simulink model "ScriptDemo"  (R2022b)
settings: configuration reference "TmVcThermal_Configuration_sub" (kept outside this file)
undefined symbols (not defined in the file): aaaa, bbbb, cTmComprCtrl_D_u8HvacFlowTable_db, cTmComprCtrl_D_u8HvacFlowTable_sw, cTmComprCtrl_n_i16ChillCmpIMax, cTmComprCtrl_n_i16ChillCmpIMin, cTmComprCtrl_n_i16ChillCmpIMin666, cTmComprCtrl_n_i16ChillCmpPMax, cTmComprCtrl_n_i16ChillCmpPMin, cTmComprCtrl_n_i16CmpChillCoolRpmKiMax, cTmComprCtrl_n_i16CmpChillCoolRpmKiMin, cTmComprCtrl_n_i16CmpChillCoolRpmKpMax, cTmComprCtrl_n_i16CmpChillCoolRpmKpMin, cTmComprCtrl_n_i16CmpCoolRpmKiMax, cTmComprCtrl_n_i16CmpCoolRpmKiMin, cTmComprCtrl_n_i16CmpCoolRpmKpMax, cTmComprCtrl_n_i16CmpCoolRpmKpMin, cTmComprCtrl_n_i16SM4CmpHeatKiMax, cTmComprCtrl_n_i16SM4CmpHeatKiMin, cTmComprCtrl_n_i16SM4CmpHeatKpMax, cTmComprCtrl_n_i16SM4CmpHeatKpMin, cTmComprCtrl_n_i16SM5CmpHeatKiMax, cTmComprCtrl_n_i16SM5CmpHeatKiMin, cTmComprCtrl_n_i16SM5CmpHeatKpMax, cTmComprCtrl_n_i16SM5CmpHeatKpMin, cTmComprCtrl_n_i16SM6CmpHeatKiMax, cTmComprCtrl_n_i16SM6CmpHeatKiMin, cTmComprCtrl_n_i16SM6CmpHeatKpMax, cTmComprCtrl_n_i16SM6CmpHeatKpMin, cTmComprCtrl_n_u16CmpMaxSpdFanFltLimt, cTmComprCtrl_n_u16CmpMaxSpdLoSidePFltLimt, cTmComprCtrl_n_u16CmpMaxSpdSensorFltLimt, cTmComprCtrl_n_u16CompMinRpm, cTmComprCtrl_n_u16CompRpmIncThres, cTmComprCtrl_t_u16BattCooltFFPeriod, cTmComprCtrl_t_u16BattCooltPIPeriod, cTmComprCtrl_t_u16CmpCoolFFPeriod, cTmComprCtrl_t_u16CmpCoolPIPeriod, cTmComprCtrl_t_u16CoolCmpChillFFPeriod, cTmComprCtrl_t_u16CoolCmpChillPIPeriod, cTmComprCtrl_t_u16SM4CmpHeatFFPeriod, cTmComprCtrl_t_u16SM4CmpHeatPIPeriod, cTmComprCtrl_t_u16SM5CmpHeatFFPeriod, cTmComprCtrl_t_u16SM5CmpHeatPIPeriod, cTmComprCtrl_t_u16SM6CmpHeatFFPeriod, cTmComprCtrl_t_u16SM6CmpHeatPIPeriod, cTmComprCtrl_Te_EvapClearInteg, cTmComprCtrl_Te_i16HpReqTempSaturoffset, cTmComprCtrl_Te_i16SatLpReplaceDiff, cTmComprCtrl_Te_i16SM3BatDiffStartEvapDecOffset, cTmComprCtrl_Te_i16SM3EvapLo, cTmComprCtrl_Te_i16SM3TBatDiffEntEvapDecOffset, cTmComprCtrl_Te_i16SM3TBatDiffEntEvapDecOffsetQuit, cTmComprCtrl_Te_s32ErrCmpChillPIContinueCoolH, cTmComprCtrl_Te_s32ErrCmpChillPIContinueCoolL, cTmComprCtrl_Te_s32ErrCmpPIContinueChillH, cTmComprCtrl_Te_s32ErrCmpPIContinueChillL, cTmComprCtrl_Te_s32ErrCmpPIContinueCoolH, cTmComprCtrl_Te_s32ErrCmpPIContinueCoolL, cTmComprCtrl_Te_s32ErrCmpPIContinueHeatH ... (+398)
libraries: simulink x782, PCMULib x640, simulink_need_slupdate x4
(part 12 of 41)

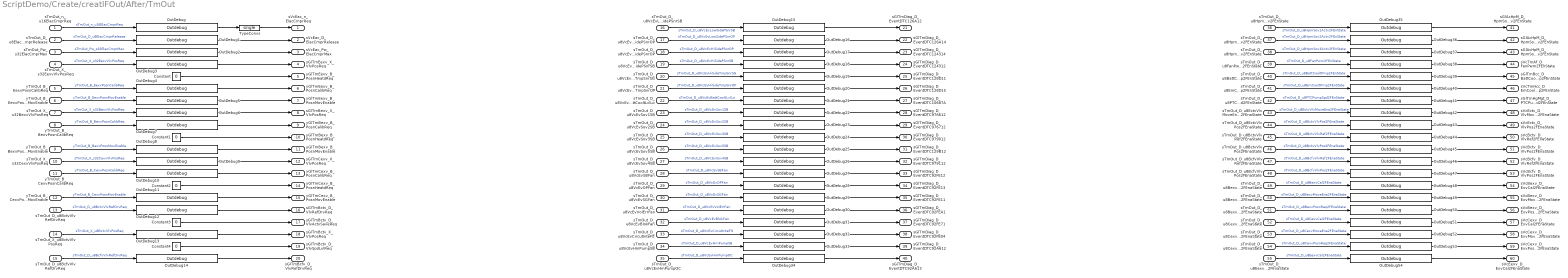
== system ScriptDemo/Create/creatIFOut/After/TmOut ==
  sTmOut_n_u16ElacCmprReq : Inport  OutDataTypeStr=uint16
  sTmOut_D_u8ElacCmprRelease : Inport  Port=2  OutDataTypeStr=uint8
  sTmOut_Pw_s32ElacCmprMax : Inport  Port=3  OutDataTypeStr=single
  sTmOut_X_s32EexvVlvPosReq : Inport  Port=4  OutDataTypeStr=single
  yTmOut_B_EexvPosnCalibReq : Inport  Port=5  OutDataTypeStr=boolean
  yTmOut_B_EexvPosnMovEnable : Inport  Port=6  OutDataTypeStr=boolean
  sTmOut_X_s32BexvVlvPosReq : Inport  Port=7  OutDataTypeStr=single
  yTmOut_B_BexvPosnCalibReq : Inport  Port=8  OutDataTypeStr=boolean
  yTmOut_B_BexvPosnMovEnable : Inport  Port=9  OutDataTypeStr=boolean
  sTmOut_X_s32CexvVlvPosReq : Inport  Port=10  OutDataTypeStr=single
  yTmOut_B_CexvPosnCalibReq : Inport  Port=11  OutDataTypeStr=boolean
  yTmOut_B_CexvPosnMovEnable : Inport  Port=12  OutDataTypeStr=boolean
  sTmOut_D_u8BctvVlvRefDrvReq : Inport  Port=13  OutDataTypeStr=uint8
  sTmOut_X_u8BctvVlvPosReq : Inport  Port=14  OutDataTypeStr=uint8
  sTmOut_D_u8BcfvVlvRefDrvReq : Inport  Port=15  OutDataTypeStr=uint8
  sTmOut_D_u8VcEvLowSidePSnrSB : Inport  Port=16  OutDataTypeStr=uint8
  sTmOut_D_u8VcEvLowSidePSnrOP : Inport  Port=17  OutDataTypeStr=uint8
  sTmOut_D_u8VcEvHiSidePSnrOP : Inport  Port=18  OutDataTypeStr=uint8
  sTmOut_D_u8VcEvHiSidePSnrSB : Inport  Port=19  OutDataTypeStr=uint8
  sTmOut_D_u8VcEvHiSideTmpSnrSG : Inport  Port=20  OutDataTypeStr=uint8
  sTmOut_D_u8VcEvHiSideTmpSnrOP : Inport  Port=21  OutDataTypeStr=uint8
  sTmOut_D_u8VcEvBattCooltLvlLo : Inport  Port=22  OutDataTypeStr=uint8
  sTmOut_D_u8VcEvSov1SB : Inport  Port=23  OutDataTypeStr=uint8
  sTmOut_D_u8VcEvSov2SB : Inport  Port=24  OutDataTypeStr=uint8
  sTmOut_D_u8VcEvSov3SB : Inport  Port=25  OutDataTypeStr=uint8
  sTmOut_D_u8VcEvSov5SB : Inport  Port=26  OutDataTypeStr=uint8
  sTmOut_D_u8VcEvSov4SB : Inport  Port=27  OutDataTypeStr=uint8
  sTmOut_D_u8VcEvSBFan : Inport  Port=28  OutDataTypeStr=uint8
  sTmOut_D_u8VcEvOPFan : Inport  Port=29  OutDataTypeStr=uint8
  sTmOut_D_u8VcEvSGFan : Inport  Port=30  OutDataTypeStr=uint8
  sTmOut_D_u8VcEvVolErrFan : Inport  Port=31  OutDataTypeStr=uint8
  sTmOut_D_u8VcEvBlokFan : Inport  Port=32  OutDataTypeStr=uint8
  sTmOut_D_u8VcEvCircutInteFlt : Inport  Port=33  OutDataTypeStr=uint8
  sTmOut_D_u8VcEvHmPumpSB : Inport  Port=34  OutDataTypeStr=uint8
  sTmOut_D_u8VcEvHmPumpOC : Inport  Port=35  OutDataTypeStr=uint8
  sTmOut_D_u8HpmSov1Actv2FEnState : Inport  Port=36  OutDataTypeStr=uint8
  sTmOut_D_u8HpmSov2Actv2FEnState : Inport  Port=37  OutDataTypeStr=uint8
  sTmOut_D_u8HpmSov3Actv2FEnState : Inport  Port=38  OutDataTypeStr=uint8
  sTmOut_D_u8FanPwm2FEnState : Inport  Port=39  OutDataTypeStr=uint8
  sTmOut_D_u8BattCooltPmp2FEnState : Inport  Port=40  OutDataTypeStr=uint8
  sTmOut_D_u8EmCooltPmp2FEnState : Inport  Port=41  OutDataTypeStr=uint8
  sTmOut_D_u8PTCPumpSpd2FEnState : Inport  Port=42  OutDataTypeStr=uint8
  sTmOut_D_u8EctvVlvMoveEna2FEnaState : Inport  Port=43  OutDataTypeStr=uint8
  sTmOut_D_u8EctvVlvPos2FEnaState : Inport  Port=44  OutDataTypeStr=uint8
  sTmOut_D_u8BctvVlvRef2FEnaState : Inport  Port=45  OutDataTypeStr=uint8
  sTmOut_D_u8BctvVlvPos2FEnaState : Inport  Port=46  OutDataTypeStr=uint8
  sTmOut_D_u8BcfvVlvRef2FEnaState : Inport  Port=47  OutDataTypeStr=uint8
  sTmOut_D_u8BcfvVlvPos2FEnaState : Inport  Port=48  OutDataTypeStr=uint8
  sTmOut_D_u8BexvCal2FEnaState : Inport  Port=49  OutDataTypeStr=uint8
  sTmOut_D_u8BexvMoveEna2FEnaState : Inport  Port=50  OutDataTypeStr=uint8
  sTmOut_D_u8BexvPosnReq2FEnaState : Inport  Port=51  OutDataTypeStr=uint8
  sTmOut_D_u8CexvCal2FEnaState : Inport  Port=52  OutDataTypeStr=uint8
  sTmOut_D_u8CexvMoveEna2FEnaState : Inport  Port=53  OutDataTypeStr=uint8
  sTmOut_D_u8CexvPosnReq2FEnaState : Inport  Port=54  OutDataTypeStr=uint8
  sTmOut_D_u8EexvCal2FEnaState : Inport  Port=55  OutDataTypeStr=uint8
  Constant : Constant  Value=0  OutDataTypeStr=boolean
  Constant1 : Constant  Value=0  OutDataTypeStr=boolean
  Constant2 : Constant  Value=0  OutDataTypeStr=boolean
  Constant3 : Constant  Value=0  OutDataTypeStr=uint8
  Constant4 : Constant  Value=0  OutDataTypeStr=uint8
  OutDebug : PCMULib/Interface/Outdebug  SWI=cTmOut_n_u16ElacCmprReq_sw  DBI=cTmOut_n_u16ElacCmprReq_db
      settings: SourceProductName=PCMULib
  OutDebug1 : PCMULib/Interface/Outdebug  SWI=cTmOut_D_u8ElacCmprRelease_sw  DBI=cTmOut_D_u8ElacCmprRelease_db
      settings: SourceProductName=PCMULib
  OutDebug10 : PCMULib/Interface/Outdebug  SWI=cTmOut_B_CexvPosnCalibReq_sw  DBI=cTmOut_B_CexvPosnCalibReq_db
      settings: SourceProductName=PCMULib
  OutDebug11 : PCMULib/Interface/Outdebug  SWI=cTmOut_B_CexvPosnMovEnable_sw  DBI=cTmOut_B_CexvPosnMovEnable_db
      settings: SourceProductName=PCMULib
  OutDebug12 : PCMULib/Interface/Outdebug  SWI=cTmOut_D_u8BctvVlvRefDrvReq_sw  DBI=cTmOut_D_u8BctvVlvRefDrvReq_db
      settings: SourceProductName=PCMULib
  OutDebug13 : PCMULib/Interface/Outdebug  SWI=cTmOut_X_u8BctvVlvPosReq_sw  DBI=cTmOut_X_u8BctvVlvPosReq_db
      settings: SourceProductName=PCMULib
  OutDebug14 : PCMULib/Interface/Outdebug  SWI=cTmOut_D_u8BcfvVlvRefDrvReq_sw  DBI=cTmOut_D_u8BcfvVlvRefDrvReq_db
      settings: SourceProductName=PCMULib
  OutDebug15 : PCMULib/Interface/Outdebug  SWI=cTmOut_D_u8VcEvLowSidePSnrSB_sw  DBI=cTmOut_D_u8VcEvLowSidePSnrSB_db
      settings: SourceProductName=PCMULib
  OutDebug16 : PCMULib/Interface/Outdebug  SWI=cTmOut_D_u8VcEvLowSidePSnrOP_sw  DBI=cTmOut_D_u8VcEvLowSidePSnrOP_db
      settings: SourceProductName=PCMULib
  OutDebug17 : PCMULib/Interface/Outdebug  SWI=cTmOut_D_u8VcEvHiSidePSnrOP_sw  DBI=cTmOut_D_u8VcEvHiSidePSnrOP_db
      settings: SourceProductName=PCMULib
  OutDebug18 : PCMULib/Interface/Outdebug  SWI=cTmOut_D_u8VcEvHiSidePSnrSB_sw  DBI=cTmOut_D_u8VcEvHiSidePSnrSB_db
      settings: SourceProductName=PCMULib
  OutDebug19 : PCMULib/Interface/Outdebug  SWI=cTmOut_D_u8VcEvHiSideTmpSnrSG_sw  DBI=cTmOut_D_u8VcEvHiSideTmpSnrSG_db
      settings: SourceProductName=PCMULib
  OutDebug2 : PCMULib/Interface/Outdebug  SWI=cTmOut_Pw_s32ElacCmprMax_sw  DBI=cTmOut_Pw_s32ElacCmprMax_db
      settings: SourceProductName=PCMULib
  OutDebug20 : PCMULib/Interface/Outdebug  SWI=cTmOut_D_u8VcEvHiSideTmpSnrOP_sw  DBI=cTmOut_D_u8VcEvHiSideTmpSnrOP_db
      settings: SourceProductName=PCMULib
  OutDebug21 : PCMULib/Interface/Outdebug  SWI=cTmOut_D_u8VcEvBattCooltLvlLo_sw  DBI=cTmOut_D_u8VcEvBattCooltLvlLo_db
      settings: SourceProductName=PCMULib
  OutDebug22 : PCMULib/Interface/Outdebug  SWI=cTmOut_D_u8VcEvSov1SB_sw  DBI=cTmOut_D_u8VcEvSov1SB_db
      settings: SourceProductName=PCMULib
  OutDebug23 : PCMULib/Interface/Outdebug  SWI=cTmOut_D_u8VcEvSov2SB_sw  DBI=cTmOut_D_u8VcEvSov2SB_db
      settings: SourceProductName=PCMULib
  OutDebug24 : PCMULib/Interface/Outdebug  SWI=cTmOut_D_u8VcEvSov3SB_sw  DBI=cTmOut_D_u8VcEvSov3SB_db
      settings: SourceProductName=PCMULib
  OutDebug25 : PCMULib/Interface/Outdebug  SWI=cTmOut_D_u8VcEvSov5SB_sw  DBI=cTmOut_D_u8VcEvSov5SB_db
      settings: SourceProductName=PCMULib
  OutDebug26 : PCMULib/Interface/Outdebug  SWI=cTmOut_D_u8VcEvSov4SB_sw  DBI=cTmOut_D_u8VcEvSov4SB_db
      settings: SourceProductName=PCMULib
  OutDebug27 : PCMULib/Interface/Outdebug  SWI=cTmOut_D_u8VcEvSBFan_sw  DBI=cTmOut_D_u8VcEvSBFan_db
      settings: SourceProductName=PCMULib
  OutDebug28 : PCMULib/Interface/Outdebug  SWI=cTmOut_D_u8VcEvOPFan_sw  DBI=cTmOut_D_u8VcEvOPFan_db
      settings: SourceProductName=PCMULib
  OutDebug29 : PCMULib/Interface/Outdebug  SWI=cTmOut_D_u8VcEvSGFan_sw  DBI=cTmOut_D_u8VcEvSGFan_db
      settings: SourceProductName=PCMULib
  OutDebug3 : PCMULib/Interface/Outdebug  SWI=cTmOut_X_s32EexvVlvPosReq_sw  DBI=cTmOut_X_s32EexvVlvPosReq_db
      settings: SourceProductName=PCMULib
  OutDebug30 : PCMULib/Interface/Outdebug  SWI=cTmOut_D_u8VcEvVolErrFan_sw  DBI=cTmOut_D_u8VcEvVolErrFan_db
      settings: SourceProductName=PCMULib
  OutDebug31 : PCMULib/Interface/Outdebug  SWI=cTmOut_D_u8VcEvBlokFan_sw  DBI=cTmOut_D_u8VcEvBlokFan_db
      settings: SourceProductName=PCMULib
  OutDebug32 : PCMULib/Interface/Outdebug  SWI=cTmOut_D_u8VcEvCircutInteFlt_sw  DBI=cTmOut_D_u8VcEvCircutInteFlt_db
      settings: SourceProductName=PCMULib
  OutDebug33 : PCMULib/Interface/Outdebug  SWI=cTmOut_D_u8VcEvHmPumpSB_sw  DBI=cTmOut_D_u8VcEvHmPumpSB_db
      settings: SourceProductName=PCMULib
  OutDebug34 : PCMULib/Interface/Outdebug  SWI=cTmOut_D_u8VcEvHmPumpOC_sw  DBI=cTmOut_D_u8VcEvHmPumpOC_db
      settings: SourceProductName=PCMULib
  OutDebug35 : PCMULib/Interface/Outdebug  SWI=cTmOut_D_u8HpmSov1Actv2FEnState_sw  DBI=cTmOut_D_u8HpmSov1Actv2FEnState_db
      settings: SourceProductName=PCMULib
  OutDebug36 : PCMULib/Interface/Outdebug  SWI=cTmOut_D_u8HpmSov2Actv2FEnState_sw  DBI=cTmOut_D_u8HpmSov2Actv2FEnState_db
      settings: SourceProductName=PCMULib
  OutDebug37 : PCMULib/Interface/Outdebug  SWI=cTmOut_D_u8HpmSov3Actv2FEnState_sw  DBI=cTmOut_D_u8HpmSov3Actv2FEnState_db
      settings: SourceProductName=PCMULib
  OutDebug38 : PCMULib/Interface/Outdebug  SWI=cTmOut_D_u8FanPwm2FEnState_sw  DBI=cTmOut_D_u8FanPwm2FEnState_db
      settings: SourceProductName=PCMULib
  OutDebug39 : PCMULib/Interface/Outdebug  SWI=cTmOut_D_u8BattCooltPmp2FEnState_sw  DBI=cTmOut_D_u8BattCooltPmp2FEnState_db
      settings: SourceProductName=PCMULib
  OutDebug4 : PCMULib/Interface/Outdebug  SWI=cTmOut_B_EexvPosnCalibReq_sw  DBI=cTmOut_B_EexvPosnCalibReq_db
      settings: SourceProductName=PCMULib
  OutDebug40 : PCMULib/Interface/Outdebug  SWI=cTmOut_D_u8EmCooltPmp2FEnState_sw  DBI=cTmOut_D_u8EmCooltPmp2FEnState_db
      settings: SourceProductName=PCMULib
  OutDebug41 : PCMULib/Interface/Outdebug  SWI=cTmOut_D_u8PTCPumpSpd2FEnState_sw  DBI=cTmOut_D_u8PTCPumpSpd2FEnState_db
      settings: SourceProductName=PCMULib
  OutDebug42 : PCMULib/Interface/Outdebug  SWI=cTmOut_D_u8EctvVlvMoveEna2FEnaState_sw  DBI=cTmOut_D_u8EctvVlvMoveEna2FEnaState_db
      settings: SourceProductName=PCMULib
  OutDebug43 : PCMULib/Interface/Outdebug  SWI=cTmOut_D_u8EctvVlvPos2FEnaState_sw  DBI=cTmOut_D_u8EctvVlvPos2FEnaState_db
      settings: SourceProductName=PCMULib
  OutDebug44 : PCMULib/Interface/Outdebug  SWI=cTmOut_D_u8BctvVlvRef2FEnaState_sw  DBI=cTmOut_D_u8BctvVlvRef2FEnaState_db
      settings: SourceProductName=PCMULib
  OutDebug45 : PCMULib/Interface/Outdebug  SWI=cTmOut_D_u8BctvVlvPos2FEnaState_sw  DBI=cTmOut_D_u8BctvVlvPos2FEnaState_db
      settings: SourceProductName=PCMULib
  OutDebug46 : PCMULib/Interface/Outdebug  SWI=cTmOut_D_u8BcfvVlvRef2FEnaState_sw  DBI=cTmOut_D_u8BcfvVlvRef2FEnaState_db
      settings: SourceProductName=PCMULib
  OutDebug47 : PCMULib/Interface/Outdebug  SWI=cTmOut_D_u8BcfvVlvPos2FEnaState_sw  DBI=cTmOut_D_u8BcfvVlvPos2FEnaState_db
      settings: SourceProductName=PCMULib
  OutDebug48 : PCMULib/Interface/Outdebug  SWI=cTmOut_D_u8BexvCal2FEnaState_sw  DBI=cTmOut_D_u8BexvCal2FEnaState_db
      settings: SourceProductName=PCMULib
  OutDebug49 : PCMULib/Interface/Outdebug  SWI=cTmOut_D_u8BexvMoveEna2FEnaState_sw  DBI=cTmOut_D_u8BexvMoveEna2FEnaState_db
      settings: SourceProductName=PCMULib
  OutDebug5 : PCMULib/Interface/Outdebug  SWI=cTmOut_B_EexvPosnMovEnable_sw  DBI=cTmOut_B_EexvPosnMovEnable_db
      settings: SourceProductName=PCMULib
  OutDebug50 : PCMULib/Interface/Outdebug  SWI=cTmOut_D_u8BexvPosnReq2FEnaState_sw  DBI=cTmOut_D_u8BexvPosnReq2FEnaState_db
      settings: SourceProductName=PCMULib
  OutDebug51 : PCMULib/Interface/Outdebug  SWI=cTmOut_D_u8CexvCal2FEnaState_sw  DBI=cTmOut_D_u8CexvCal2FEnaState_db
      settings: SourceProductName=PCMULib
  OutDebug52 : PCMULib/Interface/Outdebug  SWI=cTmOut_D_u8CexvMoveEna2FEnaState_sw  DBI=cTmOut_D_u8CexvMoveEna2FEnaState_db
      settings: SourceProductName=PCMULib
  OutDebug53 : PCMULib/Interface/Outdebug  SWI=cTmOut_D_u8CexvPosnReq2FEnaState_sw  DBI=cTmOut_D_u8CexvPosnReq2FEnaState_db
      settings: SourceProductName=PCMULib
  OutDebug54 : PCMULib/Interface/Outdebug  SWI=cTmOut_D_u8EexvCal2FEnaState_sw  DBI=cTmOut_D_u8EexvCal2FEnaState_db
      settings: SourceProductName=PCMULib
  OutDebug6 : PCMULib/Interface/Outdebug  SWI=cTmOut_X_s32BexvVlvPosReq_sw  DBI=cTmOut_X_s32BexvVlvPosReq_db
      settings: SourceProductName=PCMULib
  OutDebug7 : PCMULib/Interface/Outdebug  SWI=cTmOut_B_BexvPosnCalibReq_sw  DBI=cTmOut_B_BexvPosnCalibReq_db
      settings: SourceProductName=PCMULib
  OutDebug8 : PCMULib/Interface/Outdebug  SWI=cTmOut_B_BexvPosnMovEnable_sw  DBI=cTmOut_B_BexvPosnMovEnable_db
      settings: SourceProductName=PCMULib
  OutDebug9 : PCMULib/Interface/Outdebug  SWI=cTmOut_X_s32CexvVlvPosReq_sw  DBI=cTmOut_X_s32CexvVlvPosReq_db
      settings: SourceProductName=PCMULib
  TypeConvs : DataTypeConversion  OutDataTypeStr=single
  sVcEac_n_ElacCmprReq : Outport  OutDataTypeStr=single
  sVcEac_D_ElacCmprRelease : Outport  Port=2  OutDataTypeStr=uint8
  sVcEac_Pw_ElacCmprMax : Outport  Port=3  OutDataTypeStr=single
  sGlTmEexv_X_VlvPosReq : Outport  Port=4  OutDataTypeStr=single
  yGlTmEexv_B_PosnHeatdReq : Outport  Port=5  OutDataTypeStr=boolean
  yGlTmEexv_B_PosnCalibReq : Outport  Port=6  OutDataTypeStr=boolean
  yGlTmEexv_B_PosnMovEnable : Outport  Port=7  OutDataTypeStr=boolean
  sGlTmBexv_X_VlvPosReq : Outport  Port=8  OutDataTypeStr=single
  yGlTmBexv_B_PosnCalibReq : Outport  Port=9  OutDataTypeStr=boolean
  yGlTmBexv_B_PosnHeatdReq : Outport  Port=10  OutDataTypeStr=boolean
  yGlTmBexv_B_PosnMovEnable : Outport  Port=11  OutDataTypeStr=boolean
  sGlTmCexv_X_VlvPosReq : Outport  Port=12  OutDataTypeStr=single
  yGlTmCexv_B_PosnCalibReq : Outport  Port=13  OutDataTypeStr=boolean
  yGlTmCexv_B_PosnHeatdReq : Outport  Port=14  OutDataTypeStr=boolean
  yGlTmCexv_B_PosnMovEnable : Outport  Port=15  OutDataTypeStr=boolean
  sGlTmBctv_D_VlvRefDrvReq : Outport  Port=16  OutDataTypeStr=uint8
  sGlTmBctv_D_VlvActvSaveReq : Outport  Port=17  OutDataTypeStr=uint8
  sGlTmBctv_X_VlvPosReq : Outport  Port=18  OutDataTypeStr=uint8
  sGlTmBctv_D_VlvSpdLvlReq : Outport  Port=19  OutDataTypeStr=uint8
  sGlTmBcfv_D_VlvRefDrvReq : Outport  Port=20  OutDataTypeStr=uint8
  sGlTmDiag_D_EventDTC126A12 : Outport  Port=21  OutDataTypeStr=uint8
  sGlTmDiag_D_EventDTC126A14 : Outport  Port=22  OutDataTypeStr=uint8
  sGlTmDiag_D_EventDTC124314 : Outport  Port=23  OutDataTypeStr=uint8
  sGlTmDiag_D_EventDTC124312 : Outport  Port=24  OutDataTypeStr=uint8
  sGlTmDiag_D_EventDTC128D11 : Outport  Port=25  OutDataTypeStr=uint8
  sGlTmDiag_D_EventDTC128D15 : Outport  Port=26  OutDataTypeStr=uint8
  sGlTmDiag_D_EventDTC10687A : Outport  Port=27  OutDataTypeStr=uint8
  sGlTmDiag_D_EventDTC976612 : Outport  Port=28  OutDataTypeStr=uint8
  sGlTmDiag_D_EventDTC976712 : Outport  Port=29  OutDataTypeStr=uint8
  sGlTmDiag_D_EventDTC979012 : Outport  Port=30  OutDataTypeStr=uint8
  sGlTmDiag_D_EventDTC129B12 : Outport  Port=31  OutDataTypeStr=uint8
  sGlTmDiag_D_EventDTC979112 : Outport  Port=32  OutDataTypeStr=uint8
  sGlTmDiag_D_EventDTC92FE12 : Outport  Port=33  OutDataTypeStr=uint8
  sGlTmDiag_D_EventDTC92FE13 : Outport  Port=34  OutDataTypeStr=uint8
  sGlTmDiag_D_EventDTC92FE11 : Outport  Port=35  OutDataTypeStr=uint8
  sGlTmDiag_D_EventDTC92FEA1 : Outport  Port=36  OutDataTypeStr=uint8
  sGlTmDiag_D_EventDTC92FE71 : Outport  Port=37  OutDataTypeStr=uint8
  sGlTmDiag_D_EventDTC92FE04 : Outport  Port=38  OutDataTypeStr=uint8
  sGlTmDiag_D_EventDTC92A612 : Outport  Port=39  OutDataTypeStr=uint8
  sGlTmDiag_D_EventDTC92A613 : Outport  Port=40  OutDataTypeStr=uint8
  sGlAcHpM_D_HpmSov1Actv2FEnState : Outport  Port=41  OutDataTypeStr=uint8
  sGlAcHpM_D_HpmSov2Actv2FEnState : Outport  Port=42  OutDataTypeStr=uint8
  sGlAcHpM_D_HpmSov3Actv2FEnState : Outport  Port=43  OutDataTypeStr=uint8
  sVcTmAf_D_FanPwm2FEnState : Outport  Port=44  OutDataTypeStr=uint8
  sGlTmBcc_D_BattCooltPmp2FEnState : Outport  Port=45  OutDataTypeStr=uint8
  sVcTmHcc_D_EmCooltPmp2FEnState : Outport  Port=46  OutDataTypeStr=uint8
  sGlTmHgMgt_D_PTCPumpSpd2FEnState : Outport  Port=47  OutDataTypeStr=uint8
  sVcEctv_D_VlvMoveEna2FEnaState : Outport  Port=48  OutDataTypeStr=uint8
  sVcEctv_D_VlvPos2FEnaState : Outport  Port=49  OutDataTypeStr=uint8
  sVcBctv_D_VlvRef2FEnaState : Outport  Port=50  OutDataTypeStr=uint8
  sVcBctv_D_VlvPos2FEnaState : Outport  Port=51  OutDataTypeStr=uint8
  sVcBcfv_D_VlvRef2FEnaState : Outport  Port=52  OutDataTypeStr=uint8
  sVcBcfv_D_VlvPos2FEnaState : Outport  Port=53  OutDataTypeStr=uint8
  sVcBexv_D_ExvCal2FEnaState : Outport  Port=54  OutDataTypeStr=uint8
  sVcBexv_D_ExvMoveEna2FEnaState : Outport  Port=55  OutDataTypeStr=uint8
  sVcBexv_D_ExvPosnReq2FEnaState : Outport  Port=56  OutDataTypeStr=uint8
  sVcCexv_D_ExvCal2FEnaState : Outport  Port=57  OutDataTypeStr=uint8
  sVcCexv_D_ExvMoveEna2FEnaState : Outport  Port=58  OutDataTypeStr=uint8
  sVcCexv_D_ExvPosnReq2FEnaState : Outport  Port=59  OutDataTypeStr=uint8
  sVcEexv_D_ExvCal2FEnaState : Outport  Port=60  OutDataTypeStr=uint8
  wires:
  sTmOut_n_u16ElacCmprReq/1 -> OutDebug/1  "sTmOut_n_u16ElacCmprReq"
  OutDebug/1 -> TypeConvs/1
  TypeConvs/1 -> sVcEac_n_ElacCmprReq/1
  sTmOut_D_u8ElacCmprRelease/1 -> OutDebug1/1  "sTmOut_D_u8ElacCmprRelease"
  OutDebug1/1 -> sVcEac_D_ElacCmprRelease/1
  sTmOut_Pw_s32ElacCmprMax/1 -> OutDebug2/1  "sTmOut_Pw_s32ElacCmprMax"
  OutDebug2/1 -> sVcEac_Pw_ElacCmprMax/1
  sTmOut_X_s32EexvVlvPosReq/1 -> OutDebug3/1  "sTmOut_X_s32EexvVlvPosReq"
  OutDebug3/1 -> sGlTmEexv_X_VlvPosReq/1
  Constant/1 -> yGlTmEexv_B_PosnHeatdReq/1
  yTmOut_B_EexvPosnCalibReq/1 -> OutDebug4/1  "yTmOut_B_EexvPosnCalibReq"
  OutDebug4/1 -> yGlTmEexv_B_PosnCalibReq/1
  yTmOut_B_EexvPosnMovEnable/1 -> OutDebug5/1  "yTmOut_B_EexvPosnMovEnable"
  OutDebug5/1 -> yGlTmEexv_B_PosnMovEnable/1
  sTmOut_X_s32BexvVlvPosReq/1 -> OutDebug6/1  "sTmOut_X_s32BexvVlvPosReq"
  OutDebug6/1 -> sGlTmBexv_X_VlvPosReq/1
  yTmOut_B_BexvPosnCalibReq/1 -> OutDebug7/1  "yTmOut_B_BexvPosnCalibReq"
  OutDebug7/1 -> yGlTmBexv_B_PosnCalibReq/1
  Constant1/1 -> yGlTmBexv_B_PosnHeatdReq/1
  yTmOut_B_BexvPosnMovEnable/1 -> OutDebug8/1  "yTmOut_B_BexvPosnMovEnable"
  OutDebug8/1 -> yGlTmBexv_B_PosnMovEnable/1
  sTmOut_X_s32CexvVlvPosReq/1 -> OutDebug9/1  "sTmOut_X_s32CexvVlvPosReq"
  OutDebug9/1 -> sGlTmCexv_X_VlvPosReq/1
  yTmOut_B_CexvPosnCalibReq/1 -> OutDebug10/1  "yTmOut_B_CexvPosnCalibReq"
  OutDebug10/1 -> yGlTmCexv_B_PosnCalibReq/1
  Constant2/1 -> yGlTmCexv_B_PosnHeatdReq/1
  yTmOut_B_CexvPosnMovEnable/1 -> OutDebug11/1  "yTmOut_B_CexvPosnMovEnable"
  OutDebug11/1 -> yGlTmCexv_B_PosnMovEnable/1
  sTmOut_D_u8BctvVlvRefDrvReq/1 -> OutDebug12/1  "sTmOut_D_u8BctvVlvRefDrvReq"
  OutDebug12/1 -> sGlTmBctv_D_VlvRefDrvReq/1
  Constant3/1 -> sGlTmBctv_D_VlvActvSaveReq/1
  sTmOut_X_u8BctvVlvPosReq/1 -> OutDebug13/1  "sTmOut_X_u8BctvVlvPosReq"
  OutDebug13/1 -> sGlTmBctv_X_VlvPosReq/1
  Constant4/1 -> sGlTmBctv_D_VlvSpdLvlReq/1
  sTmOut_D_u8BcfvVlvRefDrvReq/1 -> OutDebug14/1  "sTmOut_D_u8BcfvVlvRefDrvReq"
  OutDebug14/1 -> sGlTmBcfv_D_VlvRefDrvReq/1
  sTmOut_D_u8VcEvLowSidePSnrSB/1 -> OutDebug15/1  "sTmOut_D_u8VcEvLowSidePSnrSB"
  OutDebug15/1 -> sGlTmDiag_D_EventDTC126A12/1
  sTmOut_D_u8VcEvLowSidePSnrOP/1 -> OutDebug16/1  "sTmOut_D_u8VcEvLowSidePSnrOP"
  OutDebug16/1 -> sGlTmDiag_D_EventDTC126A14/1
  sTmOut_D_u8VcEvHiSidePSnrOP/1 -> OutDebug17/1  "sTmOut_D_u8VcEvHiSidePSnrOP"
  OutDebug17/1 -> sGlTmDiag_D_EventDTC124314/1
  sTmOut_D_u8VcEvHiSidePSnrSB/1 -> OutDebug18/1  "sTmOut_D_u8VcEvHiSidePSnrSB"
  OutDebug18/1 -> sGlTmDiag_D_EventDTC124312/1
  sTmOut_D_u8VcEvHiSideTmpSnrSG/1 -> OutDebug19/1  "sTmOut_D_u8VcEvHiSideTmpSnrSG"
  OutDebug19/1 -> sGlTmDiag_D_EventDTC128D11/1
  sTmOut_D_u8VcEvHiSideTmpSnrOP/1 -> OutDebug20/1  "sTmOut_D_u8VcEvHiSideTmpSnrOP"
  OutDebug20/1 -> sGlTmDiag_D_EventDTC128D15/1
  sTmOut_D_u8VcEvBattCooltLvlLo/1 -> OutDebug21/1  "sTmOut_D_u8VcEvBattCooltLvlLo"
  OutDebug21/1 -> sGlTmDiag_D_EventDTC10687A/1
  sTmOut_D_u8VcEvSov1SB/1 -> OutDebug22/1  "sTmOut_D_u8VcEvSov1SB"
  OutDebug22/1 -> sGlTmDiag_D_EventDTC976612/1
  sTmOut_D_u8VcEvSov2SB/1 -> OutDebug23/1  "sTmOut_D_u8VcEvSov2SB"
  OutDebug23/1 -> sGlTmDiag_D_EventDTC976712/1
  sTmOut_D_u8VcEvSov3SB/1 -> OutDebug24/1  "sTmOut_D_u8VcEvSov3SB"
  OutDebug24/1 -> sGlTmDiag_D_EventDTC979012/1
  sTmOut_D_u8VcEvSov5SB/1 -> OutDebug25/1  "sTmOut_D_u8VcEvSov5SB"
  OutDebug25/1 -> sGlTmDiag_D_EventDTC129B12/1
  sTmOut_D_u8VcEvSov4SB/1 -> OutDebug26/1  "sTmOut_D_u8VcEvSov4SB"
  OutDebug26/1 -> sGlTmDiag_D_EventDTC979112/1
  sTmOut_D_u8VcEvSBFan/1 -> OutDebug27/1  "sTmOut_D_u8VcEvSBFan"
  OutDebug27/1 -> sGlTmDiag_D_EventDTC92FE12/1
  sTmOut_D_u8VcEvOPFan/1 -> OutDebug28/1  "sTmOut_D_u8VcEvOPFan"
  OutDebug28/1 -> sGlTmDiag_D_EventDTC92FE13/1
  sTmOut_D_u8VcEvSGFan/1 -> OutDebug29/1  "sTmOut_D_u8VcEvSGFan"
  OutDebug29/1 -> sGlTmDiag_D_EventDTC92FE11/1
  sTmOut_D_u8VcEvVolErrFan/1 -> OutDebug30/1  "sTmOut_D_u8VcEvVolErrFan"
  OutDebug30/1 -> sGlTmDiag_D_EventDTC92FEA1/1
  sTmOut_D_u8VcEvBlokFan/1 -> OutDebug31/1  "sTmOut_D_u8VcEvBlokFan"
  OutDebug31/1 -> sGlTmDiag_D_EventDTC92FE71/1
  sTmOut_D_u8VcEvCircutInteFlt/1 -> OutDebug32/1  "sTmOut_D_u8VcEvCircutInteFlt"
  OutDebug32/1 -> sGlTmDiag_D_EventDTC92FE04/1
  sTmOut_D_u8VcEvHmPumpSB/1 -> OutDebug33/1  "sTmOut_D_u8VcEvHmPumpSB"
  OutDebug33/1 -> sGlTmDiag_D_EventDTC92A612/1
  sTmOut_D_u8VcEvHmPumpOC/1 -> OutDebug34/1  "sTmOut_D_u8VcEvHmPumpOC"
  OutDebug34/1 -> sGlTmDiag_D_EventDTC92A613/1
  sTmOut_D_u8HpmSov1Actv2FEnState/1 -> OutDebug35/1  "sTmOut_D_u8HpmSov1Actv2FEnState"
  OutDebug35/1 -> sGlAcHpM_D_HpmSov1Actv2FEnState/1
  sTmOut_D_u8HpmSov2Actv2FEnState/1 -> OutDebug36/1  "sTmOut_D_u8HpmSov2Actv2FEnState"
  OutDebug36/1 -> sGlAcHpM_D_HpmSov2Actv2FEnState/1
  sTmOut_D_u8HpmSov3Actv2FEnState/1 -> OutDebug37/1  "sTmOut_D_u8HpmSov3Actv2FEnState"
  OutDebug37/1 -> sGlAcHpM_D_HpmSov3Actv2FEnState/1
  sTmOut_D_u8FanPwm2FEnState/1 -> OutDebug38/1  "sTmOut_D_u8FanPwm2FEnState"
  OutDebug38/1 -> sVcTmAf_D_FanPwm2FEnState/1
  sTmOut_D_u8BattCooltPmp2FEnState/1 -> OutDebug39/1  "sTmOut_D_u8BattCooltPmp2FEnState"
  OutDebug39/1 -> sGlTmBcc_D_BattCooltPmp2FEnState/1
  sTmOut_D_u8EmCooltPmp2FEnState/1 -> OutDebug40/1  "sTmOut_D_u8EmCooltPmp2FEnState"
  OutDebug40/1 -> sVcTmHcc_D_EmCooltPmp2FEnState/1
  sTmOut_D_u8PTCPumpSpd2FEnState/1 -> OutDebug41/1  "sTmOut_D_u8PTCPumpSpd2FEnState"
  OutDebug41/1 -> sGlTmHgMgt_D_PTCPumpSpd2FEnState/1
  sTmOut_D_u8EctvVlvMoveEna2FEnaState/1 -> OutDebug42/1  "sTmOut_D_u8EctvVlvMoveEna2FEnaState"
  OutDebug42/1 -> sVcEctv_D_VlvMoveEna2FEnaState/1
  sTmOut_D_u8EctvVlvPos2FEnaState/1 -> OutDebug43/1  "sTmOut_D_u8EctvVlvPos2FEnaState"
  OutDebug43/1 -> sVcEctv_D_VlvPos2FEnaState/1
  sTmOut_D_u8BctvVlvRef2FEnaState/1 -> OutDebug44/1  "sTmOut_D_u8BctvVlvRef2FEnaState"
  OutDebug44/1 -> sVcBctv_D_VlvRef2FEnaState/1
  sTmOut_D_u8BctvVlvPos2FEnaState/1 -> OutDebug45/1  "sTmOut_D_u8BctvVlvPos2FEnaState"
  OutDebug45/1 -> sVcBctv_D_VlvPos2FEnaState/1
  sTmOut_D_u8BcfvVlvRef2FEnaState/1 -> OutDebug46/1  "sTmOut_D_u8BcfvVlvRef2FEnaState"
  OutDebug46/1 -> sVcBcfv_D_VlvRef2FEnaState/1
  sTmOut_D_u8BcfvVlvPos2FEnaState/1 -> OutDebug47/1  "sTmOut_D_u8BcfvVlvPos2FEnaState"
  OutDebug47/1 -> sVcBcfv_D_VlvPos2FEnaState/1
  sTmOut_D_u8BexvCal2FEnaState/1 -> OutDebug48/1  "sTmOut_D_u8BexvCal2FEnaState"
  OutDebug48/1 -> sVcBexv_D_ExvCal2FEnaState/1
  sTmOut_D_u8BexvMoveEna2FEnaState/1 -> OutDebug49/1  "sTmOut_D_u8BexvMoveEna2FEnaState"
  OutDebug49/1 -> sVcBexv_D_ExvMoveEna2FEnaState/1
  sTmOut_D_u8BexvPosnReq2FEnaState/1 -> OutDebug50/1  "sTmOut_D_u8BexvPosnReq2FEnaState"
  OutDebug50/1 -> sVcBexv_D_ExvPosnReq2FEnaState/1
  sTmOut_D_u8CexvCal2FEnaState/1 -> OutDebug51/1  "sTmOut_D_u8CexvCal2FEnaState"
  OutDebug51/1 -> sVcCexv_D_ExvCal2FEnaState/1
  sTmOut_D_u8CexvMoveEna2FEnaState/1 -> OutDebug52/1  "sTmOut_D_u8CexvMoveEna2FEnaState"
  OutDebug52/1 -> sVcCexv_D_ExvMoveEna2FEnaState/1
  sTmOut_D_u8CexvPosnReq2FEnaState/1 -> OutDebug53/1  "sTmOut_D_u8CexvPosnReq2FEnaState"
  OutDebug53/1 -> sVcCexv_D_ExvPosnReq2FEnaState/1
  sTmOut_D_u8EexvCal2FEnaState/1 -> OutDebug54/1  "sTmOut_D_u8EexvCal2FEnaState"
  OutDebug54/1 -> sVcEexv_D_ExvCal2FEnaState/1

== system ScriptDemo/Create/createMerge/After/ID29332_RpmPI ==
  note: 测试步骤：
      | 使能测试
      | 清I测试
      | 	不使能
      | 	模式切换
      | 保持I测试
      | 	上限保持
      | 	下限保持
      | 	边界限制清I保持
      | 累计限值
      | 	累计Kp, Ki 上限
      | 	累计Kp, Ki 下限
      | 正常PI测试
      | 	上升
      | 	下降
  rTmComprCtrl_Te_s32LowErrStop : Inport  OutDataTypeStr=single
  rTmComprCtrl_Te_s32TempError : Inport  Port=2  OutDataTypeStr=single
  rTmComprCtrl_Te_s32UpErrStop : Inport  Port=3  OutDataTypeStr=single
  rTmComprCtrl_n_u16ComprRpmFF : Inport  Port=4  OutDataTypeStr=uint16
  rTmComprCtrl_n_u16ComprRpmKi : Inport  Port=5  OutDataTypeStr=uint16
  rTmComprCtrl_n_u16ComprRpmKp : Inport  Port=6  OutDataTypeStr=uint16
  rTmComprCtrl_n_u16DisOverrideValue : Inport  Port=7  OutDataTypeStr=uint16
  rTmComprCtrl_n_i16KiLowLimit : Inport  Port=8  OutDataTypeStr=int16
  rTmComprCtrl_n_i16KiUpLimit : Inport  Port=9  OutDataTypeStr=int16
  rTmComprCtrl_n_i16KpLowLimit : Inport  Port=10  OutDataTypeStr=int16
  rTmComprCtrl_n_i16KpUpLimit : Inport  Port=11  OutDataTypeStr=int16
  rTmComprCtrl_t_u16PIPeriod : Inport  Port=12  OutDataTypeStr=uint16
  xTmComprCtrl_B_CompOnReqCompOn : Inport  Port=13  OutDataTypeStr=boolean
  xTmComprCtrl_B_Enable : Inport  Port=14  OutDataTypeStr=boolean
  xTmComprCtrl_B_ModeChanged : Inport  Port=15  OutDataTypeStr=boolean
  xTmComprCtrl_B_ReduceRpm : Inport  Port=16  OutDataTypeStr=boolean
  sTmRefriModeMgr_D_u8HPCurMode : Inport  Port=17  OutDataTypeStr=uint8
  sTmSigProces_Te_s32EvapFanFilter : Inport  Port=18  OutDataTypeStr=single
  yTmRefriModeMgr_B_CoolModeInCycle : Inport  Port=19  OutDataTypeStr=boolean
  yTmRefriModeMgr_B_HeatModeInCycle : Inport  Port=20  OutDataTypeStr=boolean
  ClearInteg : Subsystem  TreatAsAtomicUnit=on
  IndebugRvs : PCMULib/Interface/IndebugRvs  SWI=cTmComprCtrl_Te_s32LowErrStop_swi  DBI=cTmComprCtrl_Te_s32LowErrStop_dbi
      settings: SourceProductName=PCMULib
  IndebugRvs1 : PCMULib/Interface/IndebugRvs  SWI=cTmComprCtrl_Te_s32TempError_swi  DBI=cTmComprCtrl_Te_s32TempError_dbi
      settings: SourceProductName=PCMULib
  IndebugRvs10 : PCMULib/Interface/IndebugRvs  SWI=cTmComprCtrl_n_i16KpUpLimit_swi  DBI=cTmComprCtrl_n_i16KpUpLimit_dbi
      settings: SourceProductName=PCMULib
  IndebugRvs11 : PCMULib/Interface/IndebugRvs  SWI=cTmComprCtrl_t_u16PIPeriod_swi  DBI=cTmComprCtrl_t_u16PIPeriod_dbi
      settings: SourceProductName=PCMULib
  IndebugRvs12 : PCMULib/Interface/IndebugRvs  SWI=cTmComprCtrl_B_Enable_swi  DBI=cTmComprCtrl_B_Enable_dbi
      settings: SourceProductName=PCMULib
  IndebugRvs13 : PCMULib/Interface/IndebugRvs  SWI=cTmComprCtrl_B_ModeChanged_swi  DBI=cTmComprCtrl_B_ModeChanged_dbi
      settings: SourceProductName=PCMULib
  IndebugRvs2 : PCMULib/Interface/IndebugRvs  SWI=cTmComprCtrl_Te_s32UpErrStop_swi  DBI=cTmComprCtrl_Te_s32UpErrStop_dbi
      settings: SourceProductName=PCMULib
  IndebugRvs3 : PCMULib/Interface/IndebugRvs  SWI=cTmComprCtrl_n_u16ComprRpmFF_swi  DBI=cTmComprCtrl_n_u16ComprRpmFF_dbi
      settings: SourceProductName=PCMULib
  IndebugRvs4 : PCMULib/Interface/IndebugRvs  SWI=cTmComprCtrl_n_u16ComprRpmKi_swi  DBI=cTmComprCtrl_n_u16ComprRpmKi_dbi
      settings: SourceProductName=PCMULib
  IndebugRvs5 : PCMULib/Interface/IndebugRvs  SWI=cTmComprCtrl_n_u16ComprRpmKp_swi  DBI=cTmComprCtrl_n_u16ComprRpmKp_dbi
      settings: SourceProductName=PCMULib
  IndebugRvs6 : PCMULib/Interface/IndebugRvs  SWI=cTmComprCtrl_n_u16DisOverrideValue_swi  DBI=cTmComprCtrl_n_u16DisOverrideValue_dbi
      settings: SourceProductName=PCMULib
  IndebugRvs7 : PCMULib/Interface/IndebugRvs  SWI=cTmComprCtrl_n_i16KiLowLimit_swi  DBI=cTmComprCtrl_n_i16KiLowLimit_dbi
      settings: SourceProductName=PCMULib
  IndebugRvs8 : PCMULib/Interface/IndebugRvs  SWI=cTmComprCtrl_n_i16KiUpLimit_swi  DBI=cTmComprCtrl_n_i16KiUpLimit_dbi
      settings: SourceProductName=PCMULib
  IndebugRvs9 : PCMULib/Interface/IndebugRvs  SWI=cTmComprCtrl_n_i16KpLowLimit_swi  DBI=cTmComprCtrl_n_i16KpLowLimit_dbi
      settings: SourceProductName=PCMULib
  PIControler : Subsystem  AncestorBlock=PCMULib/Calculation/PI
  rTmComprCtrl_n_u16CompRpmReqPI : Outport  OutDataTypeStr=uint16
  wires:
  [rTmComprCtrl_t_u16PIPeriod] -> PIControler/3(rTmComprCtrl_t_u16PIPeriod)
  [rTmComprCtrl_Te_s32TempError] -> PIControler/4(rTmComprCtrl_Te_s32TempError)
  [rTmComprCtrl_n_u16ComprRpmFF] -> PIControler/5(rTmComprCtrl_n_u16ComprRpmFF)
  [rTmComprCtrl_n_u16ComprRpmKp] -> PIControler/6(rTmComprCtrl_n_u16ComprRpmKp)
  [rTmComprCtrl_n_u16ComprRpmKi] -> PIControler/7(rTmComprCtrl_n_u16ComprRpmKi)
  [rTmComprCtrl_n_i16KpLowLimit] -> PIControler/9(rTmComprCtrl_n_i16KpLowLimit)
  [rTmComprCtrl_n_i16KiUpLimit] -> PIControler/10(rTmComprCtrl_n_i16KiUpLimit)
  [rTmComprCtrl_n_i16KiLowLimit] -> PIControler/11(rTmComprCtrl_n_i16KiLowLimit)
  [rTmComprCtrl_Te_s32UpErrStop] -> PIControler/12(rTmComprCtrl_Te_s32UpErrStop)
  [rTmComprCtrl_Te_s32LowErrStop] -> PIControler/13(rTmComprCtrl_Te_s32LowErrStop)
  [rTmComprCtrl_n_u16DisOverrideValue] -> PIControler/14(rTmComprCtrl_n_u16DisOverrideValue)
  PIControler/1(rPIControler_n_u16CompRpmReq) -> [rPIControler_n_u16CompRpmReq]
  rTmComprCtrl_Te_s32LowErrStop/1 -> IndebugRvs/1
  rTmComprCtrl_Te_s32TempError/1 -> IndebugRvs1/1
  rTmComprCtrl_Te_s32UpErrStop/1 -> IndebugRvs2/1
  rTmComprCtrl_n_u16ComprRpmFF/1 -> IndebugRvs3/1
  rTmComprCtrl_n_u16ComprRpmKi/1 -> IndebugRvs4/1
  rTmComprCtrl_n_u16ComprRpmKp/1 -> IndebugRvs5/1
  rTmComprCtrl_n_u16DisOverrideValue/1 -> IndebugRvs6/1
  rTmComprCtrl_n_i16KiLowLimit/1 -> IndebugRvs7/1
  rTmComprCtrl_n_i16KiUpLimit/1 -> IndebugRvs8/1
  rTmComprCtrl_n_i16KpLowLimit/1 -> IndebugRvs9/1
  rTmComprCtrl_n_i16KpUpLimit/1 -> IndebugRvs10/1
  rTmComprCtrl_t_u16PIPeriod/1 -> IndebugRvs11/1
  xTmComprCtrl_B_CompOnReqCompOn/1 -> [xTmComprCtrl_B_CompOnReqCompOn]
  [rPIControler_n_u16CompRpmReq] -> rTmComprCtrl_n_u16CompRpmReqPI/1
  xTmComprCtrl_B_Enable/1 -> IndebugRvs12/1
  xTmComprCtrl_B_ModeChanged/1 -> IndebugRvs13/1
  IndebugRvs/1 -> [rTmComprCtrl_Te_s32LowErrStop]  "rTmComprCtrl_Te_s32LowErrStop"
  IndebugRvs1/1 -> [rTmComprCtrl_Te_s32TempError]  "rTmComprCtrl_Te_s32TempError"
  IndebugRvs2/1 -> [rTmComprCtrl_Te_s32UpErrStop]  "rTmComprCtrl_Te_s32UpErrStop"
  IndebugRvs3/1 -> [rTmComprCtrl_n_u16ComprRpmFF]  "rTmComprCtrl_n_u16ComprRpmFF"
  IndebugRvs4/1 -> [rTmComprCtrl_n_u16ComprRpmKi]  "rTmComprCtrl_n_u16ComprRpmKi"
  IndebugRvs5/1 -> [rTmComprCtrl_n_u16ComprRpmKp]  "rTmComprCtrl_n_u16ComprRpmKp"
  IndebugRvs7/1 -> [rTmComprCtrl_n_i16KiLowLimit]  "rTmComprCtrl_n_i16KiLowLimit"
  IndebugRvs6/1 -> [rTmComprCtrl_n_u16DisOverrideValue]  "rTmComprCtrl_n_u16DisOverrideValue"
  IndebugRvs8/1 -> [rTmComprCtrl_n_i16KiUpLimit]  "rTmComprCtrl_n_i16KiUpLimit"
  IndebugRvs9/1 -> [rTmComprCtrl_n_i16KpLowLimit]  "rTmComprCtrl_n_i16KpLowLimit"
  IndebugRvs11/1 -> [rTmComprCtrl_t_u16PIPeriod]  "rTmComprCtrl_t_u16PIPeriod"
  IndebugRvs10/1 -> [rTmComprCtrl_n_i16KpUpLimit]  "rTmComprCtrl_n_i16KpUpLimit"
  IndebugRvs12/1 -> [xTmComprCtrl_B_Enable]  "xTmComprCtrl_B_Enable"
  IndebugRvs13/1 -> [xTmComprCtrl_B_ModeChanged]  "xTmComprCtrl_B_ModeChanged"
  xTmComprCtrl_B_ReduceRpm/1 -> [xTmComprCtrl_B_ReduceRpm]
  [xTmComprCtrl_B_ReduceRpm] -> PIControler/15(xTmComprCtrl_B_ReduceRpm)
  [rTmComprCtrl_n_i16KpUpLimit] -> PIControler/8(rTmComprCtrl_n_i16KpUpLimit)
  [xTmComprCtrl_B_Enable] -> PIControler/1(xTmComprCtrl_B_Enable)
  PIControler/2(rPIControler_n_s32SAccmKi) -> [rPIControler_n_s32SAccmKi]
  [rPIControler_n_s32SAccmKi] -> ClearInteg/1(rPIControler_n_s32SAccmKi)
  [sTmRefriModeMgr_D_u8HPCurMode] -> ClearInteg/2(sTmRefriModeMgr_D_u8HPCurMode)
  [sTmSigProces_Te_s32EvapFanFilter] -> ClearInteg/3(sTmSigProces_Te_s32EvapFanFilter)
  [xTmComprCtrl_B_CompOnReqCompOn] -> ClearInteg/4(xTmComprCtrl_B_CompOnReqCompOn)
  [xTmComprCtrl_B_ModeChanged] -> ClearInteg/5(xTmComprCtrl_B_ModeChanged)
  ClearInteg/1(xClearInteg_B_ClearInteg) -> [xClearInteg_B_ClearInteg]
  [xClearInteg_B_ClearInteg] -> PIControler/2(xTmComprCtrl_B_ClearInteg)
  sTmRefriModeMgr_D_u8HPCurMode/1 -> [sTmRefriModeMgr_D_u8HPCurMode]
  sTmSigProces_Te_s32EvapFanFilter/1 -> [sTmSigProces_Te_s32EvapFanFilter]
  [yTmRefriModeMgr_B_CoolModeInCycle] -> ClearInteg/6(yTmRefriModeMgr_B_CoolModeInCycle)
  [yTmRefriModeMgr_B_HeatModeInCycle] -> ClearInteg/7(yTmRefriModeMgr_B_HeatModeInCycle)
  yTmRefriModeMgr_B_CoolModeInCycle/1 -> [yTmRefriModeMgr_B_CoolModeInCycle]
  yTmRefriModeMgr_B_HeatModeInCycle/1 -> [yTmRefriModeMgr_B_HeatModeInCycle]

== system ScriptDemo/Create/createMerge/After/SM0 ==
  Action Port : ActionPort
  Constant{,1..2,10} (4 alike) : Constant  Value=0  OutDataTypeStr=uint16
  Constant11 : Constant  Value=5  OutDataTypeStr=uint16
  Constant12 : Constant  Value=0  OutDataTypeStr=boolean
  Constant3 : Constant  Value=0  OutDataTypeStr=single
  Constant4 : Constant  Value=0  OutDataTypeStr=single
  Constant5 : Constant  Value=0  OutDataTypeStr=single
  Constant{6..9} (4 alike) : Constant  Value=0  OutDataTypeStr=int16
  rSM0_Te_s32TempError : Outport  OutDataTypeStr=single
  rSM0_n_u16ComprRpmFF : Outport  Port=2  OutDataTypeStr=uint16
  rSM0_n_u16DisOverrideValue : Outport  Port=3  OutDataTypeStr=uint16
  rSM0_t_u16PIPeriod : Outport  Port=4  OutDataTypeStr=uint16
  xSM0_B_Enable : Outport  Port=5  OutDataTypeStr=boolean
  rSM0_n_u16ComprRpmKp : Outport  Port=6  OutDataTypeStr=uint16
  rSM0_n_u16ComprRpmKi : Outport  Port=7  OutDataTypeStr=uint16
  rSM0_Te_s32UpErrStop : Outport  Port=8  OutDataTypeStr=single
  rSM0_Te_s32LowErrStop : Outport  Port=9  OutDataTypeStr=single
  rSM0_n_i16KpUpLimit : Outport  Port=10  OutDataTypeStr=int16
  rSM0_n_i16KpLowLimit : Outport  Port=11  OutDataTypeStr=int16
  rSM0_n_i16KiUpLimit : Outport  Port=12  OutDataTypeStr=int16
  rSM0_n_i16KiLowLimit : Outport  Port=13  OutDataTypeStr=int16
  wires:
  Constant/1 -> [rTmComprCtrl_n_u16ComprRpmFF]
  Constant1/1 -> [rTmComprCtrl_n_u16ComprRpmKp]
  Constant2/1 -> [rTmComprCtrl_n_u16ComprRpmKi]
  Constant4/1 -> [rTmComprCtrl_Te_s32TempError]
  Constant3/1 -> [rTmComprCtrl_Te_s32UpErrStop]
  Constant5/1 -> [rTmComprCtrl_Te_s32LowErrStop]
  Constant6/1 -> [rTmComprCtrl_n_i16KpUpLimit]
  Constant7/1 -> [rTmComprCtrl_n_i16KpLowLimit]
  Constant8/1 -> [rTmComprCtrl_n_i16KiUpLimit]
  Constant9/1 -> [rTmComprCtrl_n_i16KiLowLimit]
  Constant10/1 -> [rTmComprCtrl_n_u16DisOverrideValue]
  Constant11/1 -> [rTmComprCtrl_t_u16PIPeriod]
  Constant12/1 -> [xTmComprCtrl_B_Enable]
  [rTmComprCtrl_Te_s32TempError] -> rSM0_Te_s32TempError/1
  [rTmComprCtrl_n_u16ComprRpmFF] -> rSM0_n_u16ComprRpmFF/1
  [rTmComprCtrl_n_u16DisOverrideValue] -> rSM0_n_u16DisOverrideValue/1
  [rTmComprCtrl_t_u16PIPeriod] -> rSM0_t_u16PIPeriod/1
  [xTmComprCtrl_B_Enable] -> xSM0_B_Enable/1
  [rTmComprCtrl_n_u16ComprRpmKp] -> rSM0_n_u16ComprRpmKp/1
  [rTmComprCtrl_n_u16ComprRpmKi] -> rSM0_n_u16ComprRpmKi/1
  [rTmComprCtrl_Te_s32UpErrStop] -> rSM0_Te_s32UpErrStop/1
  [rTmComprCtrl_Te_s32LowErrStop] -> rSM0_Te_s32LowErrStop/1
  [rTmComprCtrl_n_i16KpUpLimit] -> rSM0_n_i16KpUpLimit/1
  [rTmComprCtrl_n_i16KpLowLimit] -> rSM0_n_i16KpLowLimit/1
  [rTmComprCtrl_n_i16KiUpLimit] -> rSM0_n_i16KiUpLimit/1
  [rTmComprCtrl_n_i16KiLowLimit] -> rSM0_n_i16KiLowLimit/1

== system ScriptDemo/Create/createMerge/After/SM1SM21 ==
  sTmIn_D_u8DCChrgSt : Inport  OutDataTypeStr=uint8
  sTmIn_Te_s32HvBattCooltTReq : Inport  Port=2  OutDataTypeStr=single
  sTmSigProces_D_u8BattThermReq : Inport  Port=3  OutDataTypeStr=uint8
  sTmSigProces_D_u8HvBattCoolgReq : Inport  Port=4  OutDataTypeStr=uint8
  sTmSigProces_Te_s32HvBattCooltTFilter : Inport  Port=5  OutDataTypeStr=single
  xTmComprCtrl_B_CompOnReqCompOn : Inport  Port=6  OutDataTypeStr=boolean
  sTmSigProces_Te_s32TAmb : Inport  Port=7  OutDataTypeStr=single
  sTmIn_D_u8HeatPump : Inport  Port=8  OutDataTypeStr=uint8
  Action Port : ActionPort
  Constant : Constant  Value=cTmComprCtrl_n_i16ChillCmpPMax  OutDataTypeStr=int16
  Constant1 : Constant  Value=cTmComprCtrl_t_u16BattCooltPIPeriod  OutDataTypeStr=uint16
  Constant10 : Constant  Value=0  OutDataTypeStr=uint16
  Constant12 : Constant  OutDataTypeStr=boolean
  Constant2 : Constant  Value=cTmComprCtrl_n_i16ChillCmpPMin  OutDataTypeStr=int16
  Constant3 : Constant  Value=cTmComprCtrl_Te_s32ErrCmpPIContinueChillH  OutDataTypeStr=single
  Constant4 : Constant  Value=cTmComprCtrl_n_i16ChillCmpIMax  OutDataTypeStr=int16
  Constant5 : Constant  Value=cTmComprCtrl_Te_s32ErrCmpPIContinueChillL  OutDataTypeStr=single
  Constant6 : Constant  Value=cTmComprCtrl_n_i16ChillCmpIMin  OutDataTypeStr=int16
  ID26245_SM1FF : Subsystem
  ID26247_SM1Error : Subsystem
  SM1FFEnable : Subsystem
  SM1_Ki : Subsystem
  SM1_Kp : Subsystem
  rSM1SM21_n_u16DisOverrideValue : Outport  OutDataTypeStr=uint16
  rSM1SM21_t_u16PIPeriod : Outport  Port=2  OutDataTypeStr=uint16
  rSM1SM21_Te_s32UpErrStop : Outport  Port=3  OutDataTypeStr=single
  rSM1SM21_Te_s32LowErrStop : Outport  Port=4  OutDataTypeStr=single
  rSM1SM21_n_i16KpUpLimit : Outport  Port=5  OutDataTypeStr=int16
  rSM1SM21_n_u16ComprRpmFF : Outport  Port=6  OutDataTypeStr=uint16
  rSM1SM21_n_u16ComprRpmKp : Outport  Port=7  OutDataTypeStr=uint16
  rSM1SM21_n_u16ComprRpmKi : Outport  Port=8  OutDataTypeStr=uint16
  rSM1SM21_n_i16KpLowLimit : Outport  Port=9  OutDataTypeStr=int16
  rSM1SM21_n_i16KiUpLimit : Outport  Port=10  OutDataTypeStr=int16
  rSM1SM21_n_i16KiLowLimit : Outport  Port=11  OutDataTypeStr=int16
  xSM1SM21_B_Enable : Outport  Port=12  OutDataTypeStr=boolean
  rSM1SM21_Te_s32TempError : Outport  Port=13  OutDataTypeStr=single
  wires:
  ID26247_SM1Error/1(rTmComprCtrl_Te_s32TempError) -> [rTmComprCtrl_Te_s32TempError]
  [sTmIn_Te_s32HvBattCooltTReq] -> ID26247_SM1Error/1(sTmIn_Te_s32HvBattCooltTReq)
  [sTmSigProces_Te_s32HvBattCooltTFilter] -> ID26247_SM1Error/2(sTmSigProces_Te_s32HvBattCooltTFilter)
  [sTmSigProces_D_u8BattThermReq] -> SM1_Kp/1(sTmSigProces_D_u8BattThermReq)
  [sTmIn_D_u8DCChrgSt] -> SM1_Kp/2(sTmIn_D_u8DCChrgSt)
  [sTmSigProces_D_u8HvBattCoolgReq] -> SM1_Kp/3(sTmSigProces_D_u8HvBattCoolgReq)
  [rTmComprCtrl_Te_s32TempError] -> SM1_Kp/4(rTmComprCtrl_Te_s32TempError)
  [sTmSigProces_D_u8BattThermReq] -> SM1_Ki/1(sTmSigProces_D_u8BattThermReq)
  [sTmIn_D_u8DCChrgSt] -> SM1_Ki/2(sTmIn_D_u8DCChrgSt)
  [sTmSigProces_D_u8HvBattCoolgReq] -> SM1_Ki/3(sTmSigProces_D_u8HvBattCoolgReq)
  [rTmComprCtrl_Te_s32TempError] -> SM1_Ki/4(rTmComprCtrl_Te_s32TempError)
  [sTmIn_Te_s32HvBattCooltTReq] -> ID26245_SM1FF/1(sTmIn_Te_s32HvBattCooltTReq)
  [sTmIn_D_u8DCChrgSt] -> ID26245_SM1FF/2(sTmIn_D_u8DCChrgSt)
  [sTmSigProces_D_u8HvBattCoolgReq] -> ID26245_SM1FF/3(sTmSigProces_D_u8HvBattCoolgReq)
  [xTmComprCtrl_B_CompOnReqCompOn] -> SM1FFEnable/1(xTmComprCtrl_B_CompOnReqCompOn)
  SM1FFEnable/1(SM1FFEnable_B_SM1FFEnable) -> [SM1FFEnable_B_SM1FFEnable]
  [SM1FFEnable_B_SM1FFEnable] -> ID26245_SM1FF/Enable
  SM1_Ki/1(SM1Ki) -> [rTmComprCtrl_n_u16ComprRpmKi]
  SM1_Kp/1(SM1Kp) -> [rTmComprCtrl_n_u16ComprRpmKp]
  ID26245_SM1FF/1(SM1FF) -> [rTmComprCtrl_n_u16ComprRpmFF]
  sTmIn_D_u8DCChrgSt/1 -> [sTmIn_D_u8DCChrgSt]
  sTmIn_Te_s32HvBattCooltTReq/1 -> [sTmIn_Te_s32HvBattCooltTReq]
  sTmSigProces_D_u8BattThermReq/1 -> [sTmSigProces_D_u8BattThermReq]
  sTmSigProces_D_u8HvBattCoolgReq/1 -> [sTmSigProces_D_u8HvBattCoolgReq]
  sTmSigProces_Te_s32HvBattCooltTFilter/1 -> [sTmSigProces_Te_s32HvBattCooltTFilter]
  xTmComprCtrl_B_CompOnReqCompOn/1 -> [xTmComprCtrl_B_CompOnReqCompOn]
  Constant10/1 -> [rTmComprCtrl_n_u16DisOverrideValue]
  Constant4/1 -> [rTmComprCtrl_n_i16KiUpLimit]
  Constant6/1 -> [rTmComprCtrl_n_i16KiLowLimit]
  Constant1/1 -> [rTmComprCtrl_t_u16PIPeriod]
  Constant5/1 -> [rTmComprCtrl_Te_s32LowErrStop]
  Constant2/1 -> [rTmComprCtrl_n_i16KpLowLimit]
  Constant/1 -> [rTmComprCtrl_n_i16KpUpLimit]
  Constant3/1 -> [rTmComprCtrl_Te_s32UpErrStop]
  Constant12/1 -> [xTmComprCtrl_B_Enable]
  [sTmSigProces_Te_s32TAmb] -> ID26245_SM1FF/4(sTmSigProces_Te_s32TAmb)
  sTmSigProces_Te_s32TAmb/1 -> [sTmSigProces_Te_s32TAmb]
  [sTmIn_D_u8HeatPump] -> ID26245_SM1FF/5(sTmIn_D_u8HeatPump)
  sTmIn_D_u8HeatPump/1 -> [sTmIn_D_u8HeatPump]
  [rTmComprCtrl_n_u16DisOverrideValue] -> rSM1SM21_n_u16DisOverrideValue/1
  [rTmComprCtrl_t_u16PIPeriod] -> rSM1SM21_t_u16PIPeriod/1
  [rTmComprCtrl_Te_s32UpErrStop] -> rSM1SM21_Te_s32UpErrStop/1
  [rTmComprCtrl_Te_s32LowErrStop] -> rSM1SM21_Te_s32LowErrStop/1
  [rTmComprCtrl_n_i16KpUpLimit] -> rSM1SM21_n_i16KpUpLimit/1
  [rTmComprCtrl_n_u16ComprRpmFF] -> rSM1SM21_n_u16ComprRpmFF/1
  [rTmComprCtrl_n_u16ComprRpmKp] -> rSM1SM21_n_u16ComprRpmKp/1
  [rTmComprCtrl_n_u16ComprRpmKi] -> rSM1SM21_n_u16ComprRpmKi/1
  [rTmComprCtrl_n_i16KpLowLimit] -> rSM1SM21_n_i16KpLowLimit/1
  [rTmComprCtrl_n_i16KiUpLimit] -> rSM1SM21_n_i16KiUpLimit/1
  [rTmComprCtrl_n_i16KiLowLimit] -> rSM1SM21_n_i16KiLowLimit/1
  [xTmComprCtrl_B_Enable] -> xSM1SM21_B_Enable/1
  [rTmComprCtrl_Te_s32TempError] -> rSM1SM21_Te_s32TempError/1
